simulink model "test_winds"  (R2014b)
settings: Solver=ode45  StartTime=0.0  StopTime=10.0  RelTol=1e-3
values from neighbouring files (symbols this model uses):
  TestInputs =     [unit_test_inputs.mat]
libraries: simulink_extras x10, simulink x2, csu_afm_aerodynamics_lib x1
settings Model: Creator=gnc  LastModifiedBy=mstewart
settings DebuggingCC: UnderspecifiedInitializationDetection=Classic  MergeDetectMultiDrivingBlocksExec=none  SolverPrmCheckMsg=none

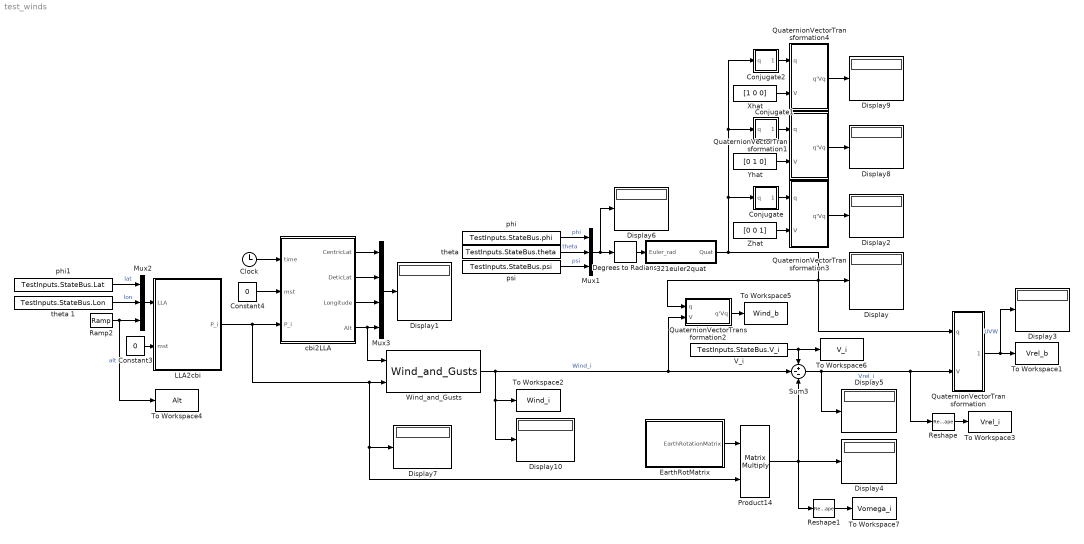
== system test_winds ==
  321euler2quat : Subsystem
  Clock : Clock
  Conjugate : Subsystem
  Conjugate1 : Subsystem
  Conjugate2 : Subsystem
  Constant3 : Constant  Value=0
  Constant4 : Constant  Value=0
  Degrees to Radians : simulink_extras/Transformations/Degrees to Radians
  Display{,1..10} (11 alike) : Display
  EarthRotMatrix : Subsystem
  LLA2cbi : Subsystem  mask(LLA to ECI Conversion){a=6378137.0, flatten=1/298.257223563}
      mask prompts: a "Central Body Semi-major Axis, a [m]"; flatten "Central Body Flattening Parameter, flatten [ND]"
      mask help: Converts Geodetic Latitude, Longitude, and Altitude into Central Body Inertial Coordinates. Inputs are [deg deg m]. Output is in [m]eters.
  Mux1 : Mux  Inputs=3
  Mux2 : Mux  Inputs=3
  Mux3 : Mux
  Product14 : Product  Multiplication=Matrix(*)  SaturateOnIntegerOverflow=on  OutDataTypeStr=Inherit: Same as first input
  QuaternionVectorTransformation : Subsystem
  QuaternionVectorTransformation1 : Subsystem
  QuaternionVectorTransformation2 : Subsystem
  QuaternionVectorTransformation3 : Subsystem
  QuaternionVectorTransformation4 : Subsystem
  Ramp2 : simulink/Sources/Ramp  slope=TestInputs.StateBus.AltDot  start=0  X0=TestInputs.StateBus.Alt
  Reshape : Reshape
  Reshape1 : Reshape
  Sum3 : Sum  Inputs=+--
  To Workspace1 : ToWorkspace  VariableName=Vrel_b  SaveFormat=Timeseries  SampleTime=-1
  To Workspace2 : ToWorkspace  VariableName=Wind_i  SaveFormat=Timeseries  SampleTime=-1
  To Workspace3 : ToWorkspace  VariableName=Vrel_i  SaveFormat=Timeseries  SampleTime=-1
  To Workspace4 : ToWorkspace  VariableName=Alt  SaveFormat=Timeseries  SampleTime=-1
  To Workspace5 : ToWorkspace  VariableName=Wind_b  SaveFormat=Timeseries  SampleTime=-1
  To Workspace6 : ToWorkspace  VariableName=V_i  SaveFormat=Timeseries  SampleTime=-1
  To Workspace7 : ToWorkspace  VariableName=Vomega_i  SaveFormat=Timeseries  SampleTime=-1
  V_i : Constant  Value=TestInputs.StateBus.V_i  VectorParams1D=off
  Wind_and_Gusts : csu_afm_aerodynamics_lib/csu_afm_aerodynamics/Wind_and_Gusts  SystemSampleTime=-1
  Xhat : Constant  Value=[1 0 0]
  Yhat : Constant  Value=[0 1 0]
  Zhat : Constant  Value=[0 0 1]
  cbi2LLA : Subsystem  mask{a=6378137.0, flatten=1/298.257223563, omega=7.2921151467e-5}
      mask prompts: a "Central Body Semi-major Axis, a [m]"; flatten "Central Body Flattening Parameter, flatten [ND]"; omega "Central Body Rotation Rate, omega [rad/s]"
      mask help:
      | % FUNCTION cbi2lla
      | %   Compute Detic Latitude, Centric Latitude, Longitude, and Detic Altitude
      | %   from Central Body Inertial Coordinates
      | %
      | %   [latD, latC, lon, alt]  = cbi2lla( P_i, mst)
      | %
      | %  INPUTS
      | %   P_i         [1x3]   {m}         Position in Central Body Inertial Frame
      | %   mst         [1x1]   (degrees)   Mean Sidereal Time
      | %
      | %  OUTPUTS
      | %   latD        [1x1]   {deg}       Detic Latitude
      | %   latC        [1x1]   {deg}       Centric Latitude
      | %   lon         [1x1]   {deg}       Longitude
      | %   alt         [1x1]   {m}         Detic Altitude
      | %
      | %  SOURCE
      | %   Borkowski, K.M. "Accurate Algorithms to Transform Geocentric to
      | %   Geodetic Coordinates"  Torun Radio Astronomy Observatory, Nicolaus
      | %   Copernicaus University, ul. Chopina 12/18, PL-87-100 Torun, Poland
      | %   Bullentin Geodesique, 63 (1989), pp. 50-56
      | %     http://www.astro.uni.torun.pl/~kb/Papers/geod/Geod-BG.htm
  phi : Constant  Value=TestInputs.StateBus.phi  VectorParams1D=off
  phi1 : Constant  Value=TestInputs.StateBus.Lat  VectorParams1D=off
  psi : Constant  Value=TestInputs.StateBus.psi  VectorParams1D=off
  "theta " : Constant  Value=TestInputs.StateBus.theta  VectorParams1D=off
  theta 1 : Constant  Value=TestInputs.StateBus.Lon  VectorParams1D=off
  wires:
  Wind_and_Gusts/1 -> Sum3/2, QuaternionVectorTransformation2/2(V), To Workspace2/1, Display10/1  "Wind_i"
  cbi2LLA/4(Alt) -> Wind_and_Gusts/1, Mux3/4
  QuaternionVectorTransformation/1(q'Vq) -> Display3/1, To Workspace1/1  "UVW"
  Sum3/1 -> Display5/1, Reshape/1, QuaternionVectorTransformation/2(V)  "Vrel_i"
  LLA2cbi/1(P_i) -> cbi2LLA/3(P_i), Wind_and_Gusts/2, Display7/1, Product14/2
  EarthRotMatrix/1(EarthRotationMatrix) -> Product14/1
  Reshape/1 -> To Workspace3/1
  phi/1 -> Mux1/1  "phi"
  "theta "/1 -> Mux1/2  "theta"
  Mux1/1 -> Display6/1, Degrees to Radians/1
  Degrees to Radians/1 -> 321euler2quat/1(Euler_rad)
  psi/1 -> Mux1/3  "psi"
  Product14/1 -> Reshape1/1, Sum3/3, Display4/1
  QuaternionVectorTransformation2/1(q'Vq) -> To Workspace5/1
  cbi2LLA/1(CentricLat) -> Mux3/1
  cbi2LLA/2(DeticLat) -> Mux3/2
  cbi2LLA/3(Longitude) -> Mux3/3
  Constant4/1 -> cbi2LLA/2(mst)
  Clock/1 -> cbi2LLA/1(time)
  Constant3/1 -> LLA2cbi/2(mst)
  Mux2/1 -> LLA2cbi/1(LLA)
  theta 1/1 -> Mux2/2  "lon"
  Ramp2/1 -> To Workspace4/1, Mux2/3  "alt"
  phi1/1 -> Mux2/1  "lat"
  Mux3/1 -> Display1/1
  Zhat/1 -> QuaternionVectorTransformation3/2(V)
  QuaternionVectorTransformation3/1(q'Vq) -> Display2/1
  V_i/1 -> To Workspace6/1, Sum3/1
  321euler2quat/1(Quat) -> Conjugate2/1(q), Conjugate1/1(q), Conjugate/1(q), QuaternionVectorTransformation/1(q), QuaternionVectorTransformation2/1(q), Display/1
  Conjugate/1(q') -> QuaternionVectorTransformation3/1(q)
  Yhat/1 -> QuaternionVectorTransformation1/2(V)
  QuaternionVectorTransformation1/1(q'Vq) -> Display8/1
  Conjugate1/1(q') -> QuaternionVectorTransformation1/1(q)
  Xhat/1 -> QuaternionVectorTransformation4/2(V)
  QuaternionVectorTransformation4/1(q'Vq) -> Display9/1
  Conjugate2/1(q') -> QuaternionVectorTransformation4/1(q)
  Reshape1/1 -> To Workspace7/1

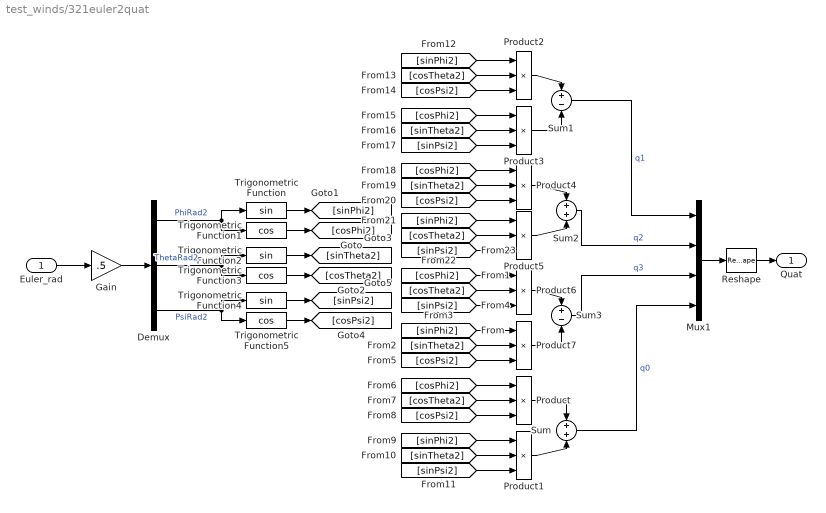
== system test_winds/321euler2quat ==
  Euler_rad : Inport
  Demux : Demux  Outputs=3
  Gain : Gain  Gain=.5
  Mux1 : Mux
  Product{,1..7} (8 alike) : Product  Inputs=3  RndMeth=Zero
  Reshape : Reshape
  Sum : Sum  Inputs=+|+
  Sum1 : Sum  Inputs=+|-
  Sum2 : Sum  Inputs=+|+
  Sum3 : Sum  Inputs=+|-
  Trigonometric Function : Trigonometry
  Trigonometric Function1 : Trigonometry  Operator=cos
  Trigonometric Function2 : Trigonometry
  Trigonometric Function3 : Trigonometry  Operator=cos
  Trigonometric Function4 : Trigonometry
  Trigonometric Function5 : Trigonometry  Operator=cos
  Quat : Outport
  wires:
  Reshape/1 -> Quat/1
  Mux1/1 -> Reshape/1
  Euler_rad/1 -> Gain/1
  [cosPsi2] -> Product7/3
  [sinTheta2] -> Product7/2
  [sinPhi2] -> Product7/1
  [sinPsi2] -> Product6/3
  [cosTheta2] -> Product6/2
  [cosPhi2] -> Product6/1
  Product6/1 -> Sum3/1
  Product7/1 -> Sum3/2
  Product5/1 -> Sum2/2
  [sinPsi2] -> Product5/3
  [cosTheta2] -> Product5/2
  [sinPhi2] -> Product5/1
  Product4/1 -> Sum2/1
  [cosPsi2] -> Product4/3
  [sinTheta2] -> Product4/2
  [cosPhi2] -> Product4/1
  Product3/1 -> Sum1/2
  [sinPsi2] -> Product3/3
  [sinTheta2] -> Product3/2
  [cosPhi2] -> Product3/1
  Product2/1 -> Sum1/1
  [cosPsi2] -> Product2/3
  [cosTheta2] -> Product2/2
  [sinPhi2] -> Product2/1
  [sinPsi2] -> Product1/3
  [sinTheta2] -> Product1/2
  [sinPhi2] -> Product1/1
  Product1/1 -> Sum/2
  Product/1 -> Sum/1
  [cosPsi2] -> Product/3
  [cosTheta2] -> Product/2
  [cosPhi2] -> Product/1
  Trigonometric Function5/1 -> [cosPsi2]
  Trigonometric Function4/1 -> [sinPsi2]
  Trigonometric Function3/1 -> [cosTheta2]
  Trigonometric Function2/1 -> [sinTheta2]
  Trigonometric Function1/1 -> [cosPhi2]
  Trigonometric Function/1 -> [sinPhi2]
  Demux/3 -> Trigonometric Function5/1, Trigonometric Function4/1  "PsiRad2"
  Demux/2 -> Trigonometric Function3/1, Trigonometric Function2/1  "ThetaRad2"
  Demux/1 -> Trigonometric Function1/1, Trigonometric Function/1  "PhiRad2"
  Gain/1 -> Demux/1
  Sum1/1 -> Mux1/1  "q1"
  Sum2/1 -> Mux1/2  "q2"
  Sum3/1 -> Mux1/3  "q3"
  Sum/1 -> Mux1/4  "q0"

== system test_winds/Conjugate ==
  q : Inport  PortDimensions=4
  Demux : Demux  Outputs=[3 1]
  Gain : Gain  Gain=-1  SaturateOnIntegerOverflow=on  OutDataTypeStr=Inherit: Same as input  ParamDataTypeStr=Inherit: Same as input
  Mux : Mux  Inputs=2
  q' : Outport  InitialOutput=0
  wires:
  Mux/1 -> q'/1
  Demux/2 -> Mux/2  "q(4)"
  Gain/1 -> Mux/1
  Demux/1 -> Gain/1  "[ q(1)  q(2)  q(3) ]"
  q/1 -> Demux/1

== system test_winds/Conjugate1 ==
  q : Inport  PortDimensions=4
  Demux : Demux  Outputs=[3 1]
  Gain : Gain  Gain=-1  SaturateOnIntegerOverflow=on  OutDataTypeStr=Inherit: Same as input  ParamDataTypeStr=Inherit: Same as input
  Mux : Mux  Inputs=2
  q' : Outport  InitialOutput=0
  wires:
  q/1 -> Demux/1
  Demux/1 -> Gain/1  "[ q(1)  q(2)  q(3) ]"
  Gain/1 -> Mux/1
  Demux/2 -> Mux/2  "q(4)"
  Mux/1 -> q'/1

== system test_winds/Conjugate2 ==
  q : Inport  PortDimensions=4
  Demux : Demux  Outputs=[3 1]
  Gain : Gain  Gain=-1  SaturateOnIntegerOverflow=on  OutDataTypeStr=Inherit: Same as input  ParamDataTypeStr=Inherit: Same as input
  Mux : Mux  Inputs=2
  q' : Outport  InitialOutput=0
  wires:
  q/1 -> Demux/1
  Demux/1 -> Gain/1  "[ q(1)  q(2)  q(3) ]"
  Gain/1 -> Mux/1
  Demux/2 -> Mux/2  "q(4)"
  Mux/1 -> q'/1

== system test_winds/EarthRotMatrix ==
  Constant{1..7} (7 alike) : Constant  Value=0
  EarthRate : Constant  Value=7.2921151467e-5
  Gain1 : Gain  Gain=-1  SaturateOnIntegerOverflow=on  OutDataTypeStr=Inherit: Same as input  ParamDataTypeStr=Inherit: Same as input
  Matrix Concatenation : Concatenate  NumInputs=3  Mode=Multidimensional array  ConcatenateDimension=2
  Mux : Mux  Inputs=3
  Mux1 : Mux  Inputs=3
  Mux2 : Mux  Inputs=3
  EarthRotationMatrix : Outport
  wires:
  Mux2/1 -> Matrix Concatenation/3
  Matrix Concatenation/1 -> EarthRotationMatrix/1
  EarthRate/1 -> [omegaE]
  [omegaE] -> Mux/2
  Constant5/1 -> Mux/1
  Constant6/1 -> Mux/3
  Constant4/1 -> Mux1/2
  Constant7/1 -> Mux2/3
  Constant3/1 -> Mux2/2
  Constant1/1 -> Mux2/1
  Constant2/1 -> Mux1/3
  Gain1/1 -> Mux1/1
  Mux1/1 -> Matrix Concatenation/2
  Mux/1 -> Matrix Concatenation/1
  [omegaE] -> Gain1/1

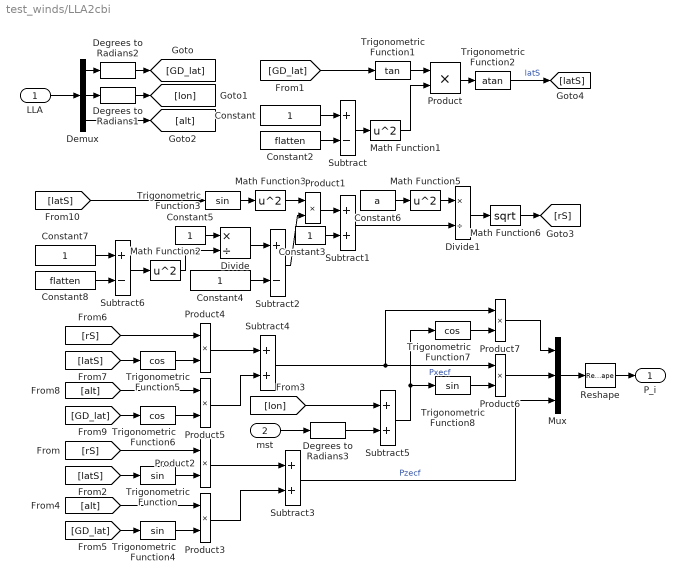
== system test_winds/LLA2cbi ==
  LLA : Inport
  mst : Inport  Port=2
  Constant{,3..5,7} (5 alike) : Constant
  Constant2 : Constant  Value=flatten
  Constant6 : Constant  Value=a
  Constant8 : Constant  Value=flatten
  Degrees to Radians1 : simulink_extras/Transformations/Degrees to Radians
  Degrees to Radians2 : simulink_extras/Transformations/Degrees to Radians
  Degrees to Radians3 : simulink_extras/Transformations/Degrees to Radians
  Demux : Demux  Outputs=3
  Divide : Product  Inputs=*/
  Divide1 : Product  Inputs=*/
  Math Function{1..3,5} (4 alike) : Math  Operator=square  SaturateOnIntegerOverflow=on
  Math Function6 : Math  Operator=sqrt  SaturateOnIntegerOverflow=on
  Mux : Mux  Inputs=3
  Product{,1..7} (8 alike) : Product  RndMeth=Zero
  Reshape : Reshape  OutputDimensionality=Column vector (2-D)
  Subtract : Sum  Inputs=+-
  Subtract{1,3..5} (4 alike) : Sum
  Subtract2 : Sum  Inputs=+-
  Subtract6 : Sum  Inputs=+-
  Trigonometric Function{,3..4,8} (4 alike) : Trigonometry
  Trigonometric Function1 : Trigonometry  Operator=tan
  Trigonometric Function2 : Trigonometry  Operator=atan
  Trigonometric Function5 : Trigonometry  Operator=cos
  Trigonometric Function6 : Trigonometry  Operator=cos
  Trigonometric Function7 : Trigonometry  Operator=cos
  P_i : Outport
  wires:
  Math Function2/1 -> Divide/2
  Subtract6/1 -> Math Function2/1
  Constant8/1 -> Subtract6/2
  Constant7/1 -> Subtract6/1
  [latS] -> Trigonometric Function3/1
  Trigonometric Function2/1 -> [latS]  "latS"
  Product6/1 -> Mux/2
  Product7/1 -> Mux/1
  Trigonometric Function7/1 -> Product7/2
  Trigonometric Function8/1 -> Product6/2
  Subtract4/1 -> Product7/1, Product6/1  "Pxecf"
  Subtract5/1 -> Trigonometric Function7/1, Trigonometric Function8/1
  [lon] -> Subtract5/1
  Degrees to Radians3/1 -> Subtract5/2
  mst/1 -> Degrees to Radians3/1
  Trigonometric Function6/1 -> Product5/2
  [alt] -> Product5/1
  Trigonometric Function5/1 -> Product4/2
  [rS] -> Product4/1
  Product5/1 -> Subtract4/2
  [GD_lat] -> Trigonometric Function6/1
  Product4/1 -> Subtract4/1
  [latS] -> Trigonometric Function5/1
  Mux/1 -> Reshape/1
  Subtract3/1 -> Mux/3  "Pzecf"
  Trigonometric Function4/1 -> Product3/2
  [alt] -> Product3/1
  Trigonometric Function/1 -> Product2/2
  [rS] -> Product2/1
  Product3/1 -> Subtract3/2
  [GD_lat] -> Trigonometric Function4/1
  Product2/1 -> Subtract3/1
  [latS] -> Trigonometric Function/1
  Math Function6/1 -> [rS]
  Divide1/1 -> Math Function6/1
  Math Function5/1 -> Divide1/1
  Subtract1/1 -> Divide1/2
  Constant6/1 -> Math Function5/1
  Product1/1 -> Subtract1/1
  Math Function3/1 -> Product1/1
  Subtract2/1 -> Product1/2
  Divide/1 -> Subtract2/1
  Constant5/1 -> Divide/1
  Constant4/1 -> Subtract2/2
  Trigonometric Function3/1 -> Math Function3/1
  Product/1 -> Trigonometric Function2/1
  Trigonometric Function1/1 -> Product/1
  [GD_lat] -> Trigonometric Function1/1
  Constant3/1 -> Subtract1/2
  Math Function1/1 -> Product/2
  Subtract/1 -> Math Function1/1
  Constant2/1 -> Subtract/2
  Constant/1 -> Subtract/1
  Degrees to Radians1/1 -> [lon]
  Degrees to Radians2/1 -> [GD_lat]
  Demux/3 -> [alt]
  Demux/2 -> Degrees to Radians1/1
  Demux/1 -> Degrees to Radians2/1
  LLA/1 -> Demux/1
  Reshape/1 -> P_i/1

== system test_winds/QuaternionVectorTransformation ==
  q : Inport  PortDimensions=4
  V : Inport  Port=2  PortDimensions=3
  Constant : Constant  Value=0
  Mux : Mux  Inputs=2
  Quaternion Conjugate : Subsystem
  Quaternion Multiply : Subsystem
  Quaternion Multiply1 : Subsystem
  Selector : Selector  InputPortWidth=4  Indices=[1 2 3]
  q'Vq : Outport  InitialOutput=0
  wires:
  Selector/1 -> q'Vq/1
  V/1 -> Mux/1
  Constant/1 -> Mux/2
  q/1 -> Quaternion Multiply1/2(q2), Quaternion Conjugate/1(q)
  Quaternion Multiply1/1(q1q2) -> Selector/1
  Mux/1 -> Quaternion Multiply/2(q2)
  Quaternion Conjugate/1(q') -> Quaternion Multiply/1(q1)
  Quaternion Multiply/1(q1q2) -> Quaternion Multiply1/1(q1)

== system test_winds/QuaternionVectorTransformation1 ==
  q : Inport  PortDimensions=4
  V : Inport  Port=2  PortDimensions=3
  Constant : Constant  Value=0
  Mux : Mux  Inputs=2
  Quaternion Conjugate : Subsystem
  Quaternion Multiply : Subsystem
  Quaternion Multiply1 : Subsystem
  Selector : Selector  InputPortWidth=4  Indices=[1 2 3]
  q'Vq : Outport  InitialOutput=0
  wires:
  Selector/1 -> q'Vq/1
  V/1 -> Mux/1
  Constant/1 -> Mux/2
  q/1 -> Quaternion Multiply1/2(q2), Quaternion Conjugate/1(q)
  Quaternion Multiply1/1(q1q2) -> Selector/1
  Mux/1 -> Quaternion Multiply/2(q2)
  Quaternion Conjugate/1(q') -> Quaternion Multiply/1(q1)
  Quaternion Multiply/1(q1q2) -> Quaternion Multiply1/1(q1)

== system test_winds/QuaternionVectorTransformation2 ==
  q : Inport  PortDimensions=4
  V : Inport  Port=2  PortDimensions=3
  Constant : Constant  Value=0
  Mux : Mux  Inputs=2
  Quaternion Conjugate : Subsystem
  Quaternion Multiply : Subsystem
  Quaternion Multiply1 : Subsystem
  Selector : Selector  InputPortWidth=4  Indices=[1 2 3]
  q'Vq : Outport  InitialOutput=0
  wires:
  Quaternion Multiply/1(q1q2) -> Quaternion Multiply1/1(q1)
  Quaternion Conjugate/1(q') -> Quaternion Multiply/1(q1)
  Mux/1 -> Quaternion Multiply/2(q2)
  Quaternion Multiply1/1(q1q2) -> Selector/1
  q/1 -> Quaternion Conjugate/1(q), Quaternion Multiply1/2(q2)
  Constant/1 -> Mux/2
  V/1 -> Mux/1
  Selector/1 -> q'Vq/1

== system test_winds/QuaternionVectorTransformation3 ==
  q : Inport  PortDimensions=4
  V : Inport  Port=2  PortDimensions=3
  Constant : Constant  Value=0
  Mux : Mux  Inputs=2
  Quaternion Conjugate : Subsystem
  Quaternion Multiply : Subsystem
  Quaternion Multiply1 : Subsystem
  Selector : Selector  InputPortWidth=4  Indices=[1 2 3]
  q'Vq : Outport  InitialOutput=0
  wires:
  Quaternion Multiply/1(q1q2) -> Quaternion Multiply1/1(q1)
  Quaternion Conjugate/1(q') -> Quaternion Multiply/1(q1)
  Mux/1 -> Quaternion Multiply/2(q2)
  Quaternion Multiply1/1(q1q2) -> Selector/1
  q/1 -> Quaternion Conjugate/1(q), Quaternion Multiply1/2(q2)
  Constant/1 -> Mux/2
  V/1 -> Mux/1
  Selector/1 -> q'Vq/1

== system test_winds/QuaternionVectorTransformation4 ==
  q : Inport  PortDimensions=4
  V : Inport  Port=2  PortDimensions=3
  Constant : Constant  Value=0
  Mux : Mux  Inputs=2
  Quaternion Conjugate : Subsystem
  Quaternion Multiply : Subsystem
  Quaternion Multiply1 : Subsystem
  Selector : Selector  InputPortWidth=4  Indices=[1 2 3]
  q'Vq : Outport  InitialOutput=0
  wires:
  Selector/1 -> q'Vq/1
  V/1 -> Mux/1
  Constant/1 -> Mux/2
  q/1 -> Quaternion Multiply1/2(q2), Quaternion Conjugate/1(q)
  Quaternion Multiply1/1(q1q2) -> Selector/1
  Mux/1 -> Quaternion Multiply/2(q2)
  Quaternion Conjugate/1(q') -> Quaternion Multiply/1(q1)
  Quaternion Multiply/1(q1q2) -> Quaternion Multiply1/1(q1)

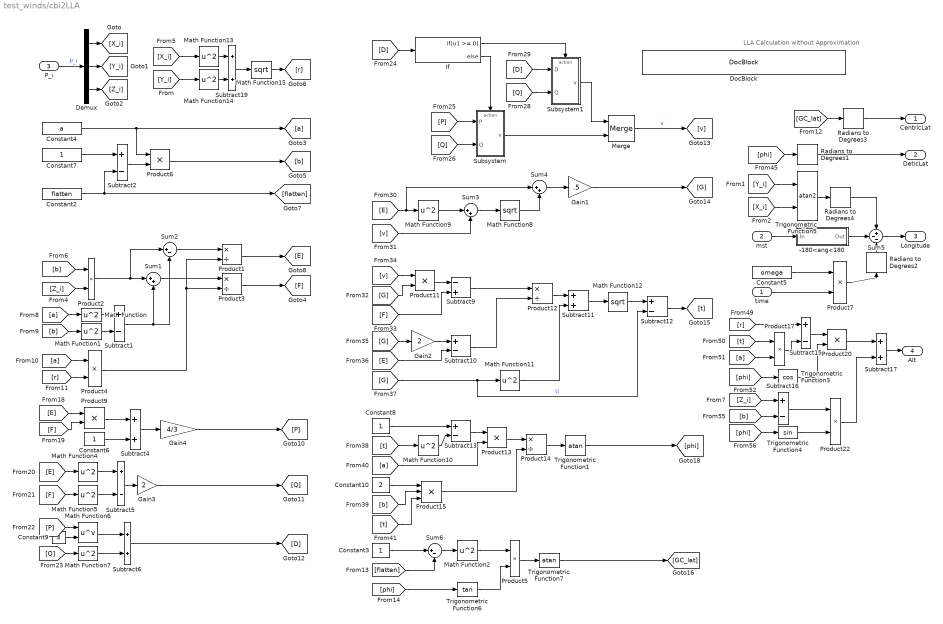
== system test_winds/cbi2LLA ==
  note: LLA Calculation without Approximation
  time : Inport
  mst : Inport  Port=2
  P_i : Inport  Port=3
  -180<ang<180 : Subsystem
  Constant10 : Constant  Value=2
  Constant2 : Constant  Value=flatten
  Constant{3,6..8} (4 alike) : Constant
  Constant4 : Constant  Value=a
  Constant5 : Constant  Value=omega
  Constant9 : Constant  Value=3
  Demux : Demux  Outputs=3
  DocBlock : simulink/Model-Wide Utilities/DocBlock  DocumentType=Text
      content=|
      | function [latD, latC, lon, alt]  = cbi2lla( P_i, mst)
      | % FUNCTION cbi2lla
      | %   Compute Detic Latitude, Centric Latitude, Longitude, and Detic Altitude
      | %   from Central Body Inertial Coordinates
      | %
      | %   [latD, latC, lon, alt]  = cbi2lla( P_i, mst)
      | %
      | %  INPUTS
      | %   P_i         [1x3]   {m}         Position in Central Body Inertial Frame
      | %   mst         [1x1]   (degrees)   Mean Sidereal Time
      | %
      | %  OUTPUTS
      | %   detic_lat   [1x1]   {deg}       Detic Latitude
      | %   centric_lat [1x1]   {deg}       Centric Latitude
      | %   lon         [1x1]   {deg}       Longitude
      | %   alt         [1x1]   {m}         Detic Altitude
      | %
      | %  SOURCE
      | %   Borkowski, K.M. "Accurate Algorithms to Transform Geocentric to
      | %   Geodetic Coordinates"  Torun Radio Astronomy Observatory, Nicolaus
      | %   Copernicaus University, ul. Chopina 12/18, PL-87-100 Torun, Poland
      | %   Bullentin Geodesique, 63 (1989), pp. 50-56
      | %     http://www.astro.uni.torun.pl/~kb/Papers/geod/Geod-BG.htm
      |
      | %% Constants
      | R2D = 180.0/acos(-1);
      | D2R = acos(-1)/180.0;
      |
      | X = P_i(1);
      | Y = P_i(2);
      | Z = P_i(3);
      |
      | %% Compute Detic Latitude & Detic Altitude ==========================
      | r = sqrt( X*X + Y*Y );
      | if (Z < 0)
      |     b = -b;
      | end
      |
      | E = ((b*Z) - (a*a - b*b))/(a*r);        % {Eq 10}
      | F = ((b*Z) + (a*a - b*b))/(a*r);        % {Eq 11}
      |
      | P = (4/3)*(E*F + 1);                    % {Eq 16}
      | Q = 2*(E*E - F*F);                      % {Eq 17}
      |
      | D = (P*P*P) + (Q*Q);                    % {Eq 15}
      | if (D < 0)
      |     v = 2*(sqrt(-P))*cos( (1/2)*acos(Q/((-P)^(3/2))) );     % {Eq 14b}
      | else
      |     v = ((sqrt(D) - Q)^(1/3)) - ((sqrt(D) + Q)^(1/3));      % {Eq 14a}
      | end
      |
      | G = (sqrt(E*E + v) + E)/2;              % {Eq 13}
      | t = sqrt( G*G + (F-v*G)/(2*G-E)) - G;   % {Eq 12}
      |
      | phi = atan( a*(1-t*t)/(2*b*t) );        % {Eq 18}
      | h = (r-a*t)*cos(phi) + (Z-b)*sin(phi);  % {Eq 19}
      |
      | latD = phi * R2D;
      | alt = h;
      |
      | %% Compute Longitude ======================================================
      | lon = atan( Y / X ) * R2D - mst;
      |
      | %% Compute Centric Latitude ============================================
      | %   Centric Latitude {deg}
      | latC = atan((1 - flatten)^2 * tan(latD * D2R)) * R2D;
  Gain1 : Gain  Gain=.5
  Gain2 : Gain  Gain=2
  Gain3 : Gain  Gain=2
  Gain4 : Gain  Gain=4/3
  If : If  IfExpression=u1 >= 0
  Math Function{,1..2,4..5,7,9..11,13..14} (11 alike) : Math  Operator=square  SaturateOnIntegerOverflow=on
  Math Function12 : Math  Operator=sqrt  SaturateOnIntegerOverflow=on
  Math Function15 : Math  Operator=sqrt  SaturateOnIntegerOverflow=on
  Math Function6 : Math  Operator=pow  SaturateOnIntegerOverflow=on
  Math Function8 : Math  Operator=sqrt  SaturateOnIntegerOverflow=on
  Merge : Merge
  Product{1,3,12,14} (4 alike) : Product  Inputs=*/  RndMeth=Zero
  Product{5..6,11,13,17,20,22} (7 alike) : Product  Inputs=**  RndMeth=Zero
  Product15 : Product  Inputs=***  RndMeth=Zero
  Product2 : Product  RndMeth=Zero
  Product4 : Product  RndMeth=Zero
  Product7 : Product  Inputs=**  SaturateOnIntegerOverflow=on  OutDataTypeStr=Inherit: Same as first input
  Product9 : Product  RndMeth=Zero
  Radians to Degrees{1..4} (4 alike) : simulink_extras/Transformations/Radians to Degrees
  Subsystem : Subsystem
  Subsystem1 : Subsystem
  Subtract{1..2,5,10,12..13,15..16} (8 alike) : Sum  Inputs=+-
  Subtract{4,6,11,17,19} (5 alike) : Sum
  Subtract9 : Sum  Inputs=-+
  Sum1 : Sum  Inputs=|++
  Sum2 : Sum  Inputs=|+-
  Sum3 : Sum  Inputs=|++
  Sum4 : Sum  Inputs=|++
  Sum5 : Sum  Inputs=+--
  Sum6 : Sum  Inputs=|+-
  Trigonometric Function1 : Trigonometry  Operator=atan
  Trigonometric Function3 : Trigonometry  Operator=cos
  Trigonometric Function4 : Trigonometry
  Trigonometric Function5 : Trigonometry  Operator=atan2
  Trigonometric Function6 : Trigonometry  Operator=tan
  Trigonometric Function7 : Trigonometry  Operator=atan
  CentricLat : Outport
  DeticLat : Outport  Port=2
  Longitude : Outport  Port=3
  Alt : Outport  Port=4
  wires:
  P_i/1 -> Demux/1  "P_i"
  [b] -> Product2/1
  [Z_i] -> Product2/2
  Product2/1 -> Sum1/1, Sum2/1
  [a] -> Math Function/1
  [b] -> Math Function1/1
  Math Function/1 -> Subtract1/1
  Math Function1/1 -> Subtract1/2
  Sum1/1 -> Product3/1
  [a] -> Product4/1
  [r] -> Product4/2
  Product4/1 -> Product3/2, Product1/2
  [E] -> Product9/1
  [F] -> Product9/2
  Constant6/1 -> Subtract4/2
  Product9/1 -> Subtract4/1
  Subtract4/1 -> Gain4/1
  [E] -> Math Function4/1
  [F] -> Math Function5/1
  Math Function4/1 -> Subtract5/1
  Math Function5/1 -> Subtract5/2
  Subtract5/1 -> Gain3/1
  Gain3/1 -> [Q]
  [P] -> Math Function6/1
  [Q] -> Math Function7/1
  Math Function6/1 -> Subtract6/1
  Math Function7/1 -> Subtract6/2
  Subtract6/1 -> [D]
  Constant9/1 -> Math Function6/2
  [D] -> If/1
  If/1 -> Subsystem1/Action
  If/2 -> Subsystem/Action
  [P] -> Subsystem/1(P)
  [Q] -> Subsystem/2(Q)
  [Q] -> Subsystem1/2(Q)
  [D] -> Subsystem1/1(D)
  Subsystem1/1(v) -> Merge/1
  Subsystem/1(v) -> Merge/2
  Merge/1 -> [v]  "v"
  [E] -> Math Function9/1, Sum4/1
  Math Function9/1 -> Sum3/1
  [v] -> Sum3/2
  Sum3/1 -> Math Function8/1
  Math Function8/1 -> Sum4/2
  Sum4/1 -> Gain1/1
  Gain1/1 -> [G]
  [G] -> Product11/2
  [v] -> Product11/1
  [F] -> Subtract9/2
  Product11/1 -> Subtract9/1
  Subtract9/1 -> Product12/1
  [G] -> Gain2/1
  Gain2/1 -> Subtract10/1
  [E] -> Subtract10/2
  Subtract10/1 -> Product12/2
  [G] -> Math Function11/1, Subtract12/2  "G"
  Product12/1 -> Subtract11/1
  Math Function11/1 -> Subtract11/2
  Subtract11/1 -> Math Function12/1
  Math Function12/1 -> Subtract12/1
  Subtract12/1 -> [t]
  [t] -> Math Function10/1
  Constant8/1 -> Subtract13/1
  Math Function10/1 -> Subtract13/2
  Subtract13/1 -> Product13/1
  [a] -> Product13/2
  Constant10/1 -> Product15/1
  [b] -> Product15/2
  [t] -> Product15/3
  Product15/1 -> Product14/2
  Product13/1 -> Product14/1
  Product14/1 -> Trigonometric Function1/1
  [phi] -> Radians to Degrees1/1
  Trigonometric Function1/1 -> [phi]
  [t] -> Product17/1
  [a] -> Product17/2
  [r] -> Subtract15/1
  Product17/1 -> Subtract15/2
  Radians to Degrees1/1 -> DeticLat/1
  [phi] -> Trigonometric Function3/1
  Subtract15/1 -> Product20/1
  Trigonometric Function3/1 -> Product20/2
  [b] -> Subtract16/2
  [Z_i] -> Subtract16/1
  [phi] -> Trigonometric Function4/1
  Subtract16/1 -> Product22/1
  Trigonometric Function4/1 -> Product22/2
  Product20/1 -> Subtract17/1
  Product22/1 -> Subtract17/2
  Subtract17/1 -> Alt/1
  Demux/1 -> [X_i]
  Demux/2 -> [Y_i]
  Demux/3 -> [Z_i]
  [X_i] -> Math Function13/1
  [Y_i] -> Math Function14/1
  Math Function13/1 -> Subtract19/1
  Math Function14/1 -> Subtract19/2
  Subtract19/1 -> Math Function15/1
  Math Function15/1 -> [r]
  Product1/1 -> [E]
  Product3/1 -> [F]
  Sum2/1 -> Product1/1
  Subtract1/1 -> Sum1/2, Sum2/2
  Gain4/1 -> [P]
  [X_i] -> Trigonometric Function5/2
  [Y_i] -> Trigonometric Function5/1
  [GC_lat] -> Radians to Degrees3/1
  Constant3/1 -> Sum6/1
  [flatten] -> Sum6/2
  Sum6/1 -> Math Function2/1
  [phi] -> Trigonometric Function6/1
  Math Function2/1 -> Product5/1
  Trigonometric Function6/1 -> Product5/2
  Product5/1 -> Trigonometric Function7/1
  Trigonometric Function7/1 -> [GC_lat]
  Radians to Degrees3/1 -> CentricLat/1
  Trigonometric Function5/1 -> Radians to Degrees4/1
  Radians to Degrees4/1 -> Sum5/1
  Sum5/1 -> Longitude/1
  Product7/1 -> Radians to Degrees2/1
  time/1 -> Product7/2
  Constant5/1 -> Product7/1
  Radians to Degrees2/1 -> Sum5/3
  mst/1 -> -180<ang<180/1(In)
  -180<ang<180/1(Out) -> Sum5/2
  Subtract2/1 -> Product6/2
  Constant2/1 -> Subtract2/2, [flatten]
  Constant7/1 -> Subtract2/1
  Constant4/1 -> Product6/1, [a]
  Product6/1 -> [b]

== system test_winds/QuaternionVectorTransformation/Quaternion Conjugate ==
  q : Inport  PortDimensions=4
  Demux : Demux  Outputs=[3 1]
  Gain : Gain  Gain=-1  SaturateOnIntegerOverflow=on  OutDataTypeStr=Inherit: Same as input  ParamDataTypeStr=Inherit: Same as input
  Mux : Mux  Inputs=2
  q' : Outport  InitialOutput=0
  wires:
  q/1 -> Demux/1
  Demux/1 -> Gain/1  "[ q(1)  q(2)  q(3) ]"
  Gain/1 -> Mux/1
  Demux/2 -> Mux/2  "q(4)"
  Mux/1 -> q'/1

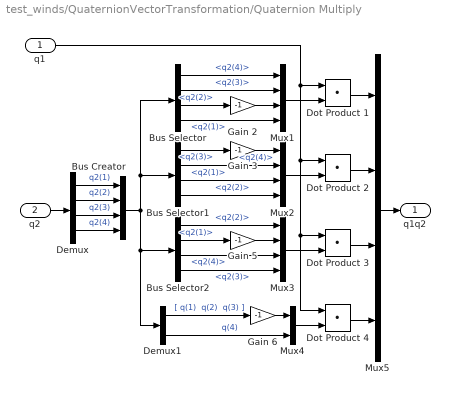
== system test_winds/QuaternionVectorTransformation/Quaternion Multiply ==
  q1 : Inport  PortDimensions=4
  q2 : Inport  Port=2  PortDimensions=4
  Bus Creator : BusCreator
  Bus Selector : BusSelector  OutputSignals=q2(4),q2(3),q2(2),q2(1)
  Bus Selector1 : BusSelector  OutputSignals=q2(3),q2(4),q2(1),q2(2)
  Bus Selector2 : BusSelector  OutputSignals=q2(2),q2(1),q2(4),q2(3)
  Demux : Demux
  Demux1 : Demux  Outputs=[3 1]
  Dot Product {1..4} (4 alike) : DotProduct  InputSameDT=on  OutDataTypeStr=Inherit: Inherit via internal rule
  Gain {2..3,5..6} (4 alike) : Gain  Gain=-1  SaturateOnIntegerOverflow=on  OutDataTypeStr=Inherit: Same as input  ParamDataTypeStr=Inherit: Same as input
  Mux{1..3,5} (4 alike) : Mux
  Mux4 : Mux  Inputs=2
  q1q2 : Outport  InitialOutput=0
  wires:
  Demux1/2 -> Mux4/2  "q(4)"
  Gain 6/1 -> Mux4/1
  Demux1/1 -> Gain 6/1  "[ q(1)  q(2)  q(3) ]"
  Mux4/1 -> Dot Product 4/2
  Bus Selector2/4 -> Mux3/4  "<q2(3)>"
  Bus Selector2/1 -> Mux3/1  "<q2(2)>"
  Gain 5/1 -> Mux3/2
  Bus Selector2/2 -> Gain 5/1  "<q2(1)>"
  Bus Selector1/4 -> Mux2/4  "<q2(2)>"
  Bus Selector1/3 -> Mux2/3  "<q2(1)>"
  Gain 3/1 -> Mux2/1
  Bus Selector1/1 -> Gain 3/1  "<q2(3)>"
  Bus Selector/4 -> Mux1/4  "<q2(1)>"
  Gain 2/1 -> Mux1/3
  Bus Selector/3 -> Gain 2/1  "<q2(2)>"
  Bus Selector/2 -> Mux1/2  "<q2(3)>"
  Bus Selector/1 -> Mux1/1  "<q2(4)>"
  Bus Selector1/2 -> Mux2/2  "<q2(4)>"
  Bus Selector2/3 -> Mux3/3  "<q2(4)>"
  Mux1/1 -> Dot Product 1/2
  Mux2/1 -> Dot Product 2/2
  Mux3/1 -> Dot Product 3/2
  q1/1 -> Dot Product 1/1, Dot Product 2/1, Dot Product 3/1, Dot Product 4/1
  Dot Product 1/1 -> Mux5/1
  Dot Product 3/1 -> Mux5/3
  Dot Product 4/1 -> Mux5/4
  Mux5/1 -> q1q2/1
  Dot Product 2/1 -> Mux5/2
  Bus Creator/1 -> Demux1/1, Bus Selector2/1, Bus Selector/1, Bus Selector1/1
  q2/1 -> Demux/1
  Demux/1 -> Bus Creator/1  "q2(1)"
  Demux/2 -> Bus Creator/2  "q2(2)"
  Demux/3 -> Bus Creator/3  "q2(3)"
  Demux/4 -> Bus Creator/4  "q2(4)"

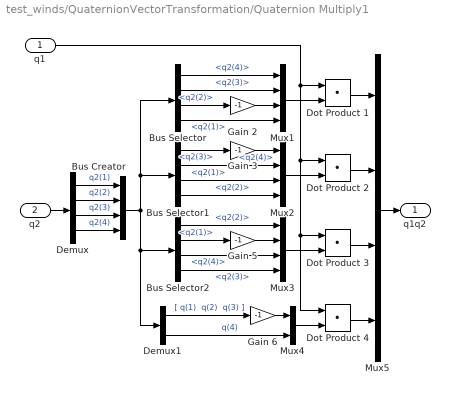
== system test_winds/QuaternionVectorTransformation/Quaternion Multiply1 ==
  q1 : Inport  PortDimensions=4
  q2 : Inport  Port=2  PortDimensions=4
  Bus Creator : BusCreator
  Bus Selector : BusSelector  OutputSignals=q2(4),q2(3),q2(2),q2(1)
  Bus Selector1 : BusSelector  OutputSignals=q2(3),q2(4),q2(1),q2(2)
  Bus Selector2 : BusSelector  OutputSignals=q2(2),q2(1),q2(4),q2(3)
  Demux : Demux
  Demux1 : Demux  Outputs=[3 1]
  Dot Product {1..4} (4 alike) : DotProduct  InputSameDT=on  OutDataTypeStr=Inherit: Inherit via internal rule
  Gain {2..3,5..6} (4 alike) : Gain  Gain=-1  SaturateOnIntegerOverflow=on  OutDataTypeStr=Inherit: Same as input  ParamDataTypeStr=Inherit: Same as input
  Mux{1..3,5} (4 alike) : Mux
  Mux4 : Mux  Inputs=2
  q1q2 : Outport  InitialOutput=0
  wires:
  Demux1/2 -> Mux4/2  "q(4)"
  Gain 6/1 -> Mux4/1
  Demux1/1 -> Gain 6/1  "[ q(1)  q(2)  q(3) ]"
  Mux4/1 -> Dot Product 4/2
  Bus Selector2/4 -> Mux3/4  "<q2(3)>"
  Bus Selector2/1 -> Mux3/1  "<q2(2)>"
  Gain 5/1 -> Mux3/2
  Bus Selector2/2 -> Gain 5/1  "<q2(1)>"
  Bus Selector1/4 -> Mux2/4  "<q2(2)>"
  Bus Selector1/3 -> Mux2/3  "<q2(1)>"
  Gain 3/1 -> Mux2/1
  Bus Selector1/1 -> Gain 3/1  "<q2(3)>"
  Bus Selector/4 -> Mux1/4  "<q2(1)>"
  Gain 2/1 -> Mux1/3
  Bus Selector/3 -> Gain 2/1  "<q2(2)>"
  Bus Selector/2 -> Mux1/2  "<q2(3)>"
  Bus Selector/1 -> Mux1/1  "<q2(4)>"
  Bus Selector1/2 -> Mux2/2  "<q2(4)>"
  Bus Selector2/3 -> Mux3/3  "<q2(4)>"
  Mux1/1 -> Dot Product 1/2
  Mux2/1 -> Dot Product 2/2
  Mux3/1 -> Dot Product 3/2
  q1/1 -> Dot Product 1/1, Dot Product 2/1, Dot Product 3/1, Dot Product 4/1
  Dot Product 1/1 -> Mux5/1
  Dot Product 3/1 -> Mux5/3
  Dot Product 4/1 -> Mux5/4
  Mux5/1 -> q1q2/1
  Dot Product 2/1 -> Mux5/2
  Bus Creator/1 -> Demux1/1, Bus Selector2/1, Bus Selector/1, Bus Selector1/1
  q2/1 -> Demux/1
  Demux/1 -> Bus Creator/1  "q2(1)"
  Demux/2 -> Bus Creator/2  "q2(2)"
  Demux/3 -> Bus Creator/3  "q2(3)"
  Demux/4 -> Bus Creator/4  "q2(4)"

== system test_winds/QuaternionVectorTransformation1/Quaternion Conjugate ==
  q : Inport  PortDimensions=4
  Demux : Demux  Outputs=[3 1]
  Gain : Gain  Gain=-1  SaturateOnIntegerOverflow=on  OutDataTypeStr=Inherit: Same as input  ParamDataTypeStr=Inherit: Same as input
  Mux : Mux  Inputs=2
  q' : Outport  InitialOutput=0
  wires:
  q/1 -> Demux/1
  Demux/1 -> Gain/1  "[ q(1)  q(2)  q(3) ]"
  Gain/1 -> Mux/1
  Demux/2 -> Mux/2  "q(4)"
  Mux/1 -> q'/1

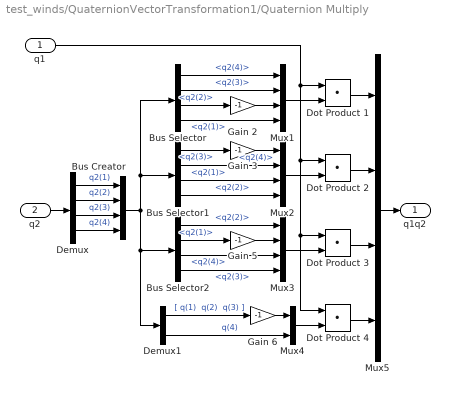
== system test_winds/QuaternionVectorTransformation1/Quaternion Multiply ==
  q1 : Inport  PortDimensions=4
  q2 : Inport  Port=2  PortDimensions=4
  Bus Creator : BusCreator
  Bus Selector : BusSelector  OutputSignals=q2(4),q2(3),q2(2),q2(1)
  Bus Selector1 : BusSelector  OutputSignals=q2(3),q2(4),q2(1),q2(2)
  Bus Selector2 : BusSelector  OutputSignals=q2(2),q2(1),q2(4),q2(3)
  Demux : Demux
  Demux1 : Demux  Outputs=[3 1]
  Dot Product {1..4} (4 alike) : DotProduct  InputSameDT=on  OutDataTypeStr=Inherit: Inherit via internal rule
  Gain {2..3,5..6} (4 alike) : Gain  Gain=-1  SaturateOnIntegerOverflow=on  OutDataTypeStr=Inherit: Same as input  ParamDataTypeStr=Inherit: Same as input
  Mux{1..3,5} (4 alike) : Mux
  Mux4 : Mux  Inputs=2
  q1q2 : Outport  InitialOutput=0
  wires:
  Demux1/2 -> Mux4/2  "q(4)"
  Gain 6/1 -> Mux4/1
  Demux1/1 -> Gain 6/1  "[ q(1)  q(2)  q(3) ]"
  Mux4/1 -> Dot Product 4/2
  Bus Selector2/4 -> Mux3/4  "<q2(3)>"
  Bus Selector2/1 -> Mux3/1  "<q2(2)>"
  Gain 5/1 -> Mux3/2
  Bus Selector2/2 -> Gain 5/1  "<q2(1)>"
  Bus Selector1/4 -> Mux2/4  "<q2(2)>"
  Bus Selector1/3 -> Mux2/3  "<q2(1)>"
  Gain 3/1 -> Mux2/1
  Bus Selector1/1 -> Gain 3/1  "<q2(3)>"
  Bus Selector/4 -> Mux1/4  "<q2(1)>"
  Gain 2/1 -> Mux1/3
  Bus Selector/3 -> Gain 2/1  "<q2(2)>"
  Bus Selector/2 -> Mux1/2  "<q2(3)>"
  Bus Selector/1 -> Mux1/1  "<q2(4)>"
  Bus Selector1/2 -> Mux2/2  "<q2(4)>"
  Bus Selector2/3 -> Mux3/3  "<q2(4)>"
  Mux1/1 -> Dot Product 1/2
  Mux2/1 -> Dot Product 2/2
  Mux3/1 -> Dot Product 3/2
  q1/1 -> Dot Product 1/1, Dot Product 2/1, Dot Product 3/1, Dot Product 4/1
  Dot Product 1/1 -> Mux5/1
  Dot Product 3/1 -> Mux5/3
  Dot Product 4/1 -> Mux5/4
  Mux5/1 -> q1q2/1
  Dot Product 2/1 -> Mux5/2
  Bus Creator/1 -> Demux1/1, Bus Selector2/1, Bus Selector/1, Bus Selector1/1
  q2/1 -> Demux/1
  Demux/1 -> Bus Creator/1  "q2(1)"
  Demux/2 -> Bus Creator/2  "q2(2)"
  Demux/3 -> Bus Creator/3  "q2(3)"
  Demux/4 -> Bus Creator/4  "q2(4)"

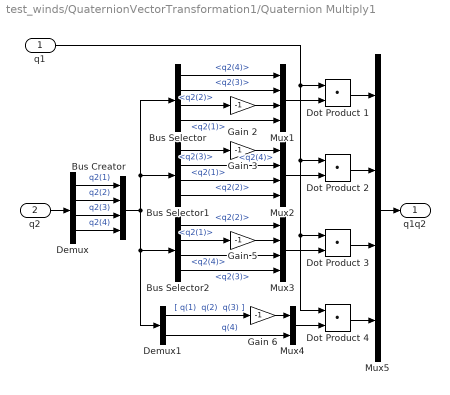
== system test_winds/QuaternionVectorTransformation1/Quaternion Multiply1 ==
  q1 : Inport  PortDimensions=4
  q2 : Inport  Port=2  PortDimensions=4
  Bus Creator : BusCreator
  Bus Selector : BusSelector  OutputSignals=q2(4),q2(3),q2(2),q2(1)
  Bus Selector1 : BusSelector  OutputSignals=q2(3),q2(4),q2(1),q2(2)
  Bus Selector2 : BusSelector  OutputSignals=q2(2),q2(1),q2(4),q2(3)
  Demux : Demux
  Demux1 : Demux  Outputs=[3 1]
  Dot Product {1..4} (4 alike) : DotProduct  InputSameDT=on  OutDataTypeStr=Inherit: Inherit via internal rule
  Gain {2..3,5..6} (4 alike) : Gain  Gain=-1  SaturateOnIntegerOverflow=on  OutDataTypeStr=Inherit: Same as input  ParamDataTypeStr=Inherit: Same as input
  Mux{1..3,5} (4 alike) : Mux
  Mux4 : Mux  Inputs=2
  q1q2 : Outport  InitialOutput=0
  wires:
  Demux1/2 -> Mux4/2  "q(4)"
  Gain 6/1 -> Mux4/1
  Demux1/1 -> Gain 6/1  "[ q(1)  q(2)  q(3) ]"
  Mux4/1 -> Dot Product 4/2
  Bus Selector2/4 -> Mux3/4  "<q2(3)>"
  Bus Selector2/1 -> Mux3/1  "<q2(2)>"
  Gain 5/1 -> Mux3/2
  Bus Selector2/2 -> Gain 5/1  "<q2(1)>"
  Bus Selector1/4 -> Mux2/4  "<q2(2)>"
  Bus Selector1/3 -> Mux2/3  "<q2(1)>"
  Gain 3/1 -> Mux2/1
  Bus Selector1/1 -> Gain 3/1  "<q2(3)>"
  Bus Selector/4 -> Mux1/4  "<q2(1)>"
  Gain 2/1 -> Mux1/3
  Bus Selector/3 -> Gain 2/1  "<q2(2)>"
  Bus Selector/2 -> Mux1/2  "<q2(3)>"
  Bus Selector/1 -> Mux1/1  "<q2(4)>"
  Bus Selector1/2 -> Mux2/2  "<q2(4)>"
  Bus Selector2/3 -> Mux3/3  "<q2(4)>"
  Mux1/1 -> Dot Product 1/2
  Mux2/1 -> Dot Product 2/2
  Mux3/1 -> Dot Product 3/2
  q1/1 -> Dot Product 1/1, Dot Product 2/1, Dot Product 3/1, Dot Product 4/1
  Dot Product 1/1 -> Mux5/1
  Dot Product 3/1 -> Mux5/3
  Dot Product 4/1 -> Mux5/4
  Mux5/1 -> q1q2/1
  Dot Product 2/1 -> Mux5/2
  Bus Creator/1 -> Demux1/1, Bus Selector2/1, Bus Selector/1, Bus Selector1/1
  q2/1 -> Demux/1
  Demux/1 -> Bus Creator/1  "q2(1)"
  Demux/2 -> Bus Creator/2  "q2(2)"
  Demux/3 -> Bus Creator/3  "q2(3)"
  Demux/4 -> Bus Creator/4  "q2(4)"

== system test_winds/QuaternionVectorTransformation2/Quaternion Conjugate ==
  q : Inport  PortDimensions=4
  Demux : Demux  Outputs=[3 1]
  Gain : Gain  Gain=-1  SaturateOnIntegerOverflow=on  OutDataTypeStr=Inherit: Same as input  ParamDataTypeStr=Inherit: Same as input
  Mux : Mux  Inputs=2
  q' : Outport  InitialOutput=0
  wires:
  Mux/1 -> q'/1
  Demux/2 -> Mux/2  "q(4)"
  Gain/1 -> Mux/1
  Demux/1 -> Gain/1  "[ q(1)  q(2)  q(3) ]"
  q/1 -> Demux/1

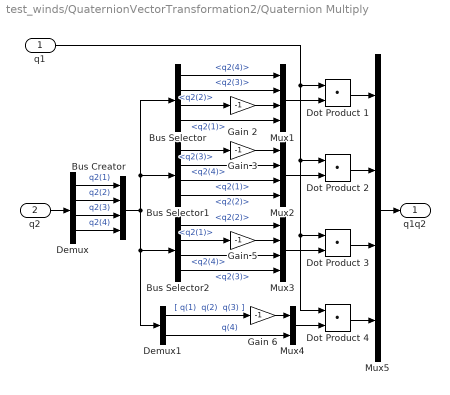
== system test_winds/QuaternionVectorTransformation2/Quaternion Multiply ==
  q1 : Inport  PortDimensions=4
  q2 : Inport  Port=2  PortDimensions=4
  Bus Creator : BusCreator
  Bus Selector : BusSelector  OutputSignals=q2(4),q2(3),q2(2),q2(1)
  Bus Selector1 : BusSelector  OutputSignals=q2(3),q2(4),q2(1),q2(2)
  Bus Selector2 : BusSelector  OutputSignals=q2(2),q2(1),q2(4),q2(3)
  Demux : Demux
  Demux1 : Demux  Outputs=[3 1]
  Dot Product {1..4} (4 alike) : DotProduct  InputSameDT=on  OutDataTypeStr=Inherit: Inherit via internal rule
  Gain {2..3,5..6} (4 alike) : Gain  Gain=-1  SaturateOnIntegerOverflow=on  OutDataTypeStr=Inherit: Same as input  ParamDataTypeStr=Inherit: Same as input
  Mux{1..3,5} (4 alike) : Mux
  Mux4 : Mux  Inputs=2
  q1q2 : Outport  InitialOutput=0
  wires:
  Demux/4 -> Bus Creator/4  "q2(4)"
  Demux/3 -> Bus Creator/3  "q2(3)"
  Demux/2 -> Bus Creator/2  "q2(2)"
  Demux/1 -> Bus Creator/1  "q2(1)"
  q2/1 -> Demux/1
  Bus Creator/1 -> Bus Selector1/1, Bus Selector/1, Bus Selector2/1, Demux1/1
  Dot Product 2/1 -> Mux5/2
  Mux5/1 -> q1q2/1
  Dot Product 4/1 -> Mux5/4
  Dot Product 3/1 -> Mux5/3
  Dot Product 1/1 -> Mux5/1
  q1/1 -> Dot Product 4/1, Dot Product 3/1, Dot Product 2/1, Dot Product 1/1
  Mux3/1 -> Dot Product 3/2
  Mux2/1 -> Dot Product 2/2
  Mux1/1 -> Dot Product 1/2
  Bus Selector2/3 -> Mux3/3  "<q2(4)>"
  Bus Selector1/2 -> Mux2/2  "<q2(4)>"
  Bus Selector/1 -> Mux1/1  "<q2(4)>"
  Bus Selector/2 -> Mux1/2  "<q2(3)>"
  Bus Selector/3 -> Gain 2/1  "<q2(2)>"
  Gain 2/1 -> Mux1/3
  Bus Selector/4 -> Mux1/4  "<q2(1)>"
  Bus Selector1/1 -> Gain 3/1  "<q2(3)>"
  Gain 3/1 -> Mux2/1
  Bus Selector1/3 -> Mux2/3  "<q2(1)>"
  Bus Selector1/4 -> Mux2/4  "<q2(2)>"
  Bus Selector2/2 -> Gain 5/1  "<q2(1)>"
  Gain 5/1 -> Mux3/2
  Bus Selector2/1 -> Mux3/1  "<q2(2)>"
  Bus Selector2/4 -> Mux3/4  "<q2(3)>"
  Mux4/1 -> Dot Product 4/2
  Demux1/1 -> Gain 6/1  "[ q(1)  q(2)  q(3) ]"
  Gain 6/1 -> Mux4/1
  Demux1/2 -> Mux4/2  "q(4)"

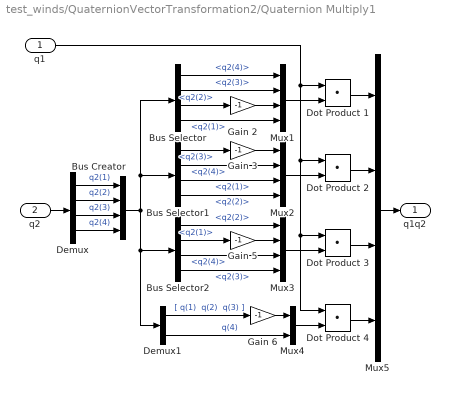
== system test_winds/QuaternionVectorTransformation2/Quaternion Multiply1 ==
  q1 : Inport  PortDimensions=4
  q2 : Inport  Port=2  PortDimensions=4
  Bus Creator : BusCreator
  Bus Selector : BusSelector  OutputSignals=q2(4),q2(3),q2(2),q2(1)
  Bus Selector1 : BusSelector  OutputSignals=q2(3),q2(4),q2(1),q2(2)
  Bus Selector2 : BusSelector  OutputSignals=q2(2),q2(1),q2(4),q2(3)
  Demux : Demux
  Demux1 : Demux  Outputs=[3 1]
  Dot Product {1..4} (4 alike) : DotProduct  InputSameDT=on  OutDataTypeStr=Inherit: Inherit via internal rule
  Gain {2..3,5..6} (4 alike) : Gain  Gain=-1  SaturateOnIntegerOverflow=on  OutDataTypeStr=Inherit: Same as input  ParamDataTypeStr=Inherit: Same as input
  Mux{1..3,5} (4 alike) : Mux
  Mux4 : Mux  Inputs=2
  q1q2 : Outport  InitialOutput=0
  wires:
  Demux/4 -> Bus Creator/4  "q2(4)"
  Demux/3 -> Bus Creator/3  "q2(3)"
  Demux/2 -> Bus Creator/2  "q2(2)"
  Demux/1 -> Bus Creator/1  "q2(1)"
  q2/1 -> Demux/1
  Bus Creator/1 -> Bus Selector1/1, Bus Selector/1, Bus Selector2/1, Demux1/1
  Dot Product 2/1 -> Mux5/2
  Mux5/1 -> q1q2/1
  Dot Product 4/1 -> Mux5/4
  Dot Product 3/1 -> Mux5/3
  Dot Product 1/1 -> Mux5/1
  q1/1 -> Dot Product 4/1, Dot Product 3/1, Dot Product 2/1, Dot Product 1/1
  Mux3/1 -> Dot Product 3/2
  Mux2/1 -> Dot Product 2/2
  Mux1/1 -> Dot Product 1/2
  Bus Selector2/3 -> Mux3/3  "<q2(4)>"
  Bus Selector1/2 -> Mux2/2  "<q2(4)>"
  Bus Selector/1 -> Mux1/1  "<q2(4)>"
  Bus Selector/2 -> Mux1/2  "<q2(3)>"
  Bus Selector/3 -> Gain 2/1  "<q2(2)>"
  Gain 2/1 -> Mux1/3
  Bus Selector/4 -> Mux1/4  "<q2(1)>"
  Bus Selector1/1 -> Gain 3/1  "<q2(3)>"
  Gain 3/1 -> Mux2/1
  Bus Selector1/3 -> Mux2/3  "<q2(1)>"
  Bus Selector1/4 -> Mux2/4  "<q2(2)>"
  Bus Selector2/2 -> Gain 5/1  "<q2(1)>"
  Gain 5/1 -> Mux3/2
  Bus Selector2/1 -> Mux3/1  "<q2(2)>"
  Bus Selector2/4 -> Mux3/4  "<q2(3)>"
  Mux4/1 -> Dot Product 4/2
  Demux1/1 -> Gain 6/1  "[ q(1)  q(2)  q(3) ]"
  Gain 6/1 -> Mux4/1
  Demux1/2 -> Mux4/2  "q(4)"

== system test_winds/QuaternionVectorTransformation3/Quaternion Conjugate ==
  q : Inport  PortDimensions=4
  Demux : Demux  Outputs=[3 1]
  Gain : Gain  Gain=-1  SaturateOnIntegerOverflow=on  OutDataTypeStr=Inherit: Same as input  ParamDataTypeStr=Inherit: Same as input
  Mux : Mux  Inputs=2
  q' : Outport  InitialOutput=0
  wires:
  Mux/1 -> q'/1
  Demux/2 -> Mux/2  "q(4)"
  Gain/1 -> Mux/1
  Demux/1 -> Gain/1  "[ q(1)  q(2)  q(3) ]"
  q/1 -> Demux/1

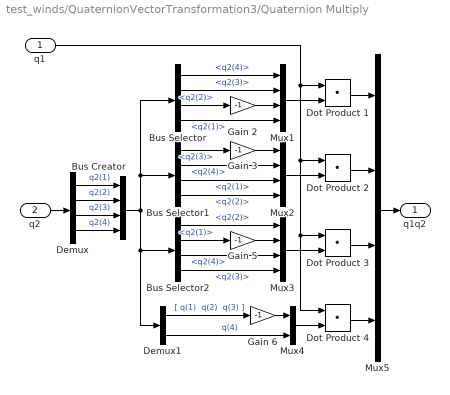
== system test_winds/QuaternionVectorTransformation3/Quaternion Multiply ==
  q1 : Inport  PortDimensions=4
  q2 : Inport  Port=2  PortDimensions=4
  Bus Creator : BusCreator
  Bus Selector : BusSelector  OutputSignals=q2(4),q2(3),q2(2),q2(1)
  Bus Selector1 : BusSelector  OutputSignals=q2(3),q2(4),q2(1),q2(2)
  Bus Selector2 : BusSelector  OutputSignals=q2(2),q2(1),q2(4),q2(3)
  Demux : Demux
  Demux1 : Demux  Outputs=[3 1]
  Dot Product {1..4} (4 alike) : DotProduct  InputSameDT=on  OutDataTypeStr=Inherit: Inherit via internal rule
  Gain {2..3,5..6} (4 alike) : Gain  Gain=-1  SaturateOnIntegerOverflow=on  OutDataTypeStr=Inherit: Same as input  ParamDataTypeStr=Inherit: Same as input
  Mux{1..3,5} (4 alike) : Mux
  Mux4 : Mux  Inputs=2
  q1q2 : Outport  InitialOutput=0
  wires:
  Demux/4 -> Bus Creator/4  "q2(4)"
  Demux/3 -> Bus Creator/3  "q2(3)"
  Demux/2 -> Bus Creator/2  "q2(2)"
  Demux/1 -> Bus Creator/1  "q2(1)"
  q2/1 -> Demux/1
  Bus Creator/1 -> Bus Selector1/1, Bus Selector/1, Bus Selector2/1, Demux1/1
  Dot Product 2/1 -> Mux5/2
  Mux5/1 -> q1q2/1
  Dot Product 4/1 -> Mux5/4
  Dot Product 3/1 -> Mux5/3
  Dot Product 1/1 -> Mux5/1
  q1/1 -> Dot Product 4/1, Dot Product 3/1, Dot Product 2/1, Dot Product 1/1
  Mux3/1 -> Dot Product 3/2
  Mux2/1 -> Dot Product 2/2
  Mux1/1 -> Dot Product 1/2
  Bus Selector2/3 -> Mux3/3  "<q2(4)>"
  Bus Selector1/2 -> Mux2/2  "<q2(4)>"
  Bus Selector/1 -> Mux1/1  "<q2(4)>"
  Bus Selector/2 -> Mux1/2  "<q2(3)>"
  Bus Selector/3 -> Gain 2/1  "<q2(2)>"
  Gain 2/1 -> Mux1/3
  Bus Selector/4 -> Mux1/4  "<q2(1)>"
  Bus Selector1/1 -> Gain 3/1  "<q2(3)>"
  Gain 3/1 -> Mux2/1
  Bus Selector1/3 -> Mux2/3  "<q2(1)>"
  Bus Selector1/4 -> Mux2/4  "<q2(2)>"
  Bus Selector2/2 -> Gain 5/1  "<q2(1)>"
  Gain 5/1 -> Mux3/2
  Bus Selector2/1 -> Mux3/1  "<q2(2)>"
  Bus Selector2/4 -> Mux3/4  "<q2(3)>"
  Mux4/1 -> Dot Product 4/2
  Demux1/1 -> Gain 6/1  "[ q(1)  q(2)  q(3) ]"
  Gain 6/1 -> Mux4/1
  Demux1/2 -> Mux4/2  "q(4)"

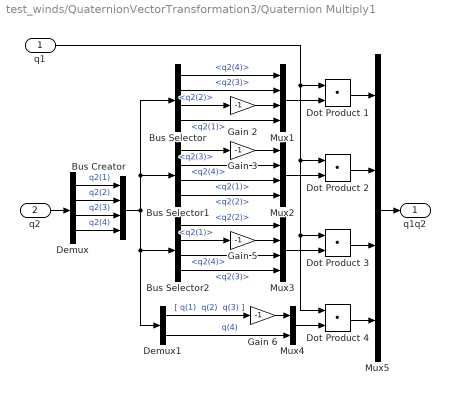
== system test_winds/QuaternionVectorTransformation3/Quaternion Multiply1 ==
  q1 : Inport  PortDimensions=4
  q2 : Inport  Port=2  PortDimensions=4
  Bus Creator : BusCreator
  Bus Selector : BusSelector  OutputSignals=q2(4),q2(3),q2(2),q2(1)
  Bus Selector1 : BusSelector  OutputSignals=q2(3),q2(4),q2(1),q2(2)
  Bus Selector2 : BusSelector  OutputSignals=q2(2),q2(1),q2(4),q2(3)
  Demux : Demux
  Demux1 : Demux  Outputs=[3 1]
  Dot Product {1..4} (4 alike) : DotProduct  InputSameDT=on  OutDataTypeStr=Inherit: Inherit via internal rule
  Gain {2..3,5..6} (4 alike) : Gain  Gain=-1  SaturateOnIntegerOverflow=on  OutDataTypeStr=Inherit: Same as input  ParamDataTypeStr=Inherit: Same as input
  Mux{1..3,5} (4 alike) : Mux
  Mux4 : Mux  Inputs=2
  q1q2 : Outport  InitialOutput=0
  wires:
  Demux/4 -> Bus Creator/4  "q2(4)"
  Demux/3 -> Bus Creator/3  "q2(3)"
  Demux/2 -> Bus Creator/2  "q2(2)"
  Demux/1 -> Bus Creator/1  "q2(1)"
  q2/1 -> Demux/1
  Bus Creator/1 -> Bus Selector1/1, Bus Selector/1, Bus Selector2/1, Demux1/1
  Dot Product 2/1 -> Mux5/2
  Mux5/1 -> q1q2/1
  Dot Product 4/1 -> Mux5/4
  Dot Product 3/1 -> Mux5/3
  Dot Product 1/1 -> Mux5/1
  q1/1 -> Dot Product 4/1, Dot Product 3/1, Dot Product 2/1, Dot Product 1/1
  Mux3/1 -> Dot Product 3/2
  Mux2/1 -> Dot Product 2/2
  Mux1/1 -> Dot Product 1/2
  Bus Selector2/3 -> Mux3/3  "<q2(4)>"
  Bus Selector1/2 -> Mux2/2  "<q2(4)>"
  Bus Selector/1 -> Mux1/1  "<q2(4)>"
  Bus Selector/2 -> Mux1/2  "<q2(3)>"
  Bus Selector/3 -> Gain 2/1  "<q2(2)>"
  Gain 2/1 -> Mux1/3
  Bus Selector/4 -> Mux1/4  "<q2(1)>"
  Bus Selector1/1 -> Gain 3/1  "<q2(3)>"
  Gain 3/1 -> Mux2/1
  Bus Selector1/3 -> Mux2/3  "<q2(1)>"
  Bus Selector1/4 -> Mux2/4  "<q2(2)>"
  Bus Selector2/2 -> Gain 5/1  "<q2(1)>"
  Gain 5/1 -> Mux3/2
  Bus Selector2/1 -> Mux3/1  "<q2(2)>"
  Bus Selector2/4 -> Mux3/4  "<q2(3)>"
  Mux4/1 -> Dot Product 4/2
  Demux1/1 -> Gain 6/1  "[ q(1)  q(2)  q(3) ]"
  Gain 6/1 -> Mux4/1
  Demux1/2 -> Mux4/2  "q(4)"

== system test_winds/QuaternionVectorTransformation4/Quaternion Conjugate ==
  q : Inport  PortDimensions=4
  Demux : Demux  Outputs=[3 1]
  Gain : Gain  Gain=-1  SaturateOnIntegerOverflow=on  OutDataTypeStr=Inherit: Same as input  ParamDataTypeStr=Inherit: Same as input
  Mux : Mux  Inputs=2
  q' : Outport  InitialOutput=0
  wires:
  q/1 -> Demux/1
  Demux/1 -> Gain/1  "[ q(1)  q(2)  q(3) ]"
  Gain/1 -> Mux/1
  Demux/2 -> Mux/2  "q(4)"
  Mux/1 -> q'/1

== system test_winds/QuaternionVectorTransformation4/Quaternion Multiply ==
  q1 : Inport  PortDimensions=4
  q2 : Inport  Port=2  PortDimensions=4
  Bus Creator : BusCreator
  Bus Selector : BusSelector  OutputSignals=q2(4),q2(3),q2(2),q2(1)
  Bus Selector1 : BusSelector  OutputSignals=q2(3),q2(4),q2(1),q2(2)
  Bus Selector2 : BusSelector  OutputSignals=q2(2),q2(1),q2(4),q2(3)
  Demux : Demux
  Demux1 : Demux  Outputs=[3 1]
  Dot Product {1..4} (4 alike) : DotProduct  InputSameDT=on  OutDataTypeStr=Inherit: Inherit via internal rule
  Gain {2..3,5..6} (4 alike) : Gain  Gain=-1  SaturateOnIntegerOverflow=on  OutDataTypeStr=Inherit: Same as input  ParamDataTypeStr=Inherit: Same as input
  Mux{1..3,5} (4 alike) : Mux
  Mux4 : Mux  Inputs=2
  q1q2 : Outport  InitialOutput=0
  wires:
  Demux1/2 -> Mux4/2  "q(4)"
  Gain 6/1 -> Mux4/1
  Demux1/1 -> Gain 6/1  "[ q(1)  q(2)  q(3) ]"
  Mux4/1 -> Dot Product 4/2
  Bus Selector2/4 -> Mux3/4  "<q2(3)>"
  Bus Selector2/1 -> Mux3/1  "<q2(2)>"
  Gain 5/1 -> Mux3/2
  Bus Selector2/2 -> Gain 5/1  "<q2(1)>"
  Bus Selector1/4 -> Mux2/4  "<q2(2)>"
  Bus Selector1/3 -> Mux2/3  "<q2(1)>"
  Gain 3/1 -> Mux2/1
  Bus Selector1/1 -> Gain 3/1  "<q2(3)>"
  Bus Selector/4 -> Mux1/4  "<q2(1)>"
  Gain 2/1 -> Mux1/3
  Bus Selector/3 -> Gain 2/1  "<q2(2)>"
  Bus Selector/2 -> Mux1/2  "<q2(3)>"
  Bus Selector/1 -> Mux1/1  "<q2(4)>"
  Bus Selector1/2 -> Mux2/2  "<q2(4)>"
  Bus Selector2/3 -> Mux3/3  "<q2(4)>"
  Mux1/1 -> Dot Product 1/2
  Mux2/1 -> Dot Product 2/2
  Mux3/1 -> Dot Product 3/2
  q1/1 -> Dot Product 1/1, Dot Product 2/1, Dot Product 3/1, Dot Product 4/1
  Dot Product 1/1 -> Mux5/1
  Dot Product 3/1 -> Mux5/3
  Dot Product 4/1 -> Mux5/4
  Mux5/1 -> q1q2/1
  Dot Product 2/1 -> Mux5/2
  Bus Creator/1 -> Demux1/1, Bus Selector2/1, Bus Selector/1, Bus Selector1/1
  q2/1 -> Demux/1
  Demux/1 -> Bus Creator/1  "q2(1)"
  Demux/2 -> Bus Creator/2  "q2(2)"
  Demux/3 -> Bus Creator/3  "q2(3)"
  Demux/4 -> Bus Creator/4  "q2(4)"

== system test_winds/QuaternionVectorTransformation4/Quaternion Multiply1 ==
  q1 : Inport  PortDimensions=4
  q2 : Inport  Port=2  PortDimensions=4
  Bus Creator : BusCreator
  Bus Selector : BusSelector  OutputSignals=q2(4),q2(3),q2(2),q2(1)
  Bus Selector1 : BusSelector  OutputSignals=q2(3),q2(4),q2(1),q2(2)
  Bus Selector2 : BusSelector  OutputSignals=q2(2),q2(1),q2(4),q2(3)
  Demux : Demux
  Demux1 : Demux  Outputs=[3 1]
  Dot Product {1..4} (4 alike) : DotProduct  InputSameDT=on  OutDataTypeStr=Inherit: Inherit via internal rule
  Gain {2..3,5..6} (4 alike) : Gain  Gain=-1  SaturateOnIntegerOverflow=on  OutDataTypeStr=Inherit: Same as input  ParamDataTypeStr=Inherit: Same as input
  Mux{1..3,5} (4 alike) : Mux
  Mux4 : Mux  Inputs=2
  q1q2 : Outport  InitialOutput=0
  wires:
  Demux1/2 -> Mux4/2  "q(4)"
  Gain 6/1 -> Mux4/1
  Demux1/1 -> Gain 6/1  "[ q(1)  q(2)  q(3) ]"
  Mux4/1 -> Dot Product 4/2
  Bus Selector2/4 -> Mux3/4  "<q2(3)>"
  Bus Selector2/1 -> Mux3/1  "<q2(2)>"
  Gain 5/1 -> Mux3/2
  Bus Selector2/2 -> Gain 5/1  "<q2(1)>"
  Bus Selector1/4 -> Mux2/4  "<q2(2)>"
  Bus Selector1/3 -> Mux2/3  "<q2(1)>"
  Gain 3/1 -> Mux2/1
  Bus Selector1/1 -> Gain 3/1  "<q2(3)>"
  Bus Selector/4 -> Mux1/4  "<q2(1)>"
  Gain 2/1 -> Mux1/3
  Bus Selector/3 -> Gain 2/1  "<q2(2)>"
  Bus Selector/2 -> Mux1/2  "<q2(3)>"
  Bus Selector/1 -> Mux1/1  "<q2(4)>"
  Bus Selector1/2 -> Mux2/2  "<q2(4)>"
  Bus Selector2/3 -> Mux3/3  "<q2(4)>"
  Mux1/1 -> Dot Product 1/2
  Mux2/1 -> Dot Product 2/2
  Mux3/1 -> Dot Product 3/2
  q1/1 -> Dot Product 1/1, Dot Product 2/1, Dot Product 3/1, Dot Product 4/1
  Dot Product 1/1 -> Mux5/1
  Dot Product 3/1 -> Mux5/3
  Dot Product 4/1 -> Mux5/4
  Mux5/1 -> q1q2/1
  Dot Product 2/1 -> Mux5/2
  Bus Creator/1 -> Demux1/1, Bus Selector2/1, Bus Selector/1, Bus Selector1/1
  q2/1 -> Demux/1
  Demux/1 -> Bus Creator/1  "q2(1)"
  Demux/2 -> Bus Creator/2  "q2(2)"
  Demux/3 -> Bus Creator/3  "q2(3)"
  Demux/4 -> Bus Creator/4  "q2(4)"

== system test_winds/cbi2LLA/-180<ang<180 ==
  In : Inport
  Degrees to Radians1 : simulink_extras/Transformations/Degrees to Radians
  Radians to Degrees : simulink_extras/Transformations/Radians to Degrees
  Trigonometric Function : Trigonometry
  Trigonometric Function1 : Trigonometry  Operator=cos
  Trigonometric Function2 : Trigonometry  Operator=atan2
  Out : Outport
  wires:
  Trigonometric Function2/1 -> Radians to Degrees/1
  In/1 -> Degrees to Radians1/1
  Trigonometric Function1/1 -> Trigonometric Function2/2
  Trigonometric Function/1 -> Trigonometric Function2/1
  Radians to Degrees/1 -> Out/1
  Degrees to Radians1/1 -> Trigonometric Function1/1, Trigonometric Function/1

== system test_winds/cbi2LLA/Subsystem ==
  P : Inport
  Q : Inport  Port=2
  Action Port : ActionPort  ActionType=else
  Constant9 : Constant  Value=3/2
  Gain1 : Gain  Gain=-1
  Gain3 : Gain  Gain=2
  Gain4 : Gain  Gain=.5
  Math Function1 : Math  Operator=sqrt  SaturateOnIntegerOverflow=on
  Math Function6 : Math  Operator=pow  SaturateOnIntegerOverflow=on
  Product1 : Product  Inputs=*/  RndMeth=Zero
  Product6 : Product  Inputs=**  RndMeth=Zero
  Trigonometric Function : Trigonometry  Operator=cos
  Trigonometric Function1 : Trigonometry  Operator=acos
  v : Outport
  wires:
  P/1 -> Gain1/1
  Gain1/1 -> Math Function1/1, Math Function6/1  "-P"
  Math Function1/1 -> Gain3/1
  Gain3/1 -> Product6/1
  Constant9/1 -> Math Function6/2
  Q/1 -> Product1/1  "Q"
  Math Function6/1 -> Product1/2
  Product1/1 -> Trigonometric Function1/1
  Trigonometric Function1/1 -> Gain4/1
  Gain4/1 -> Trigonometric Function/1
  Trigonometric Function/1 -> Product6/2
  Product6/1 -> v/1

== system test_winds/cbi2LLA/Subsystem1 ==
  D : Inport
  Q : Inport  Port=2
  Action Port : ActionPort  ActionType=then
  Constant2 : Constant  Value=1/3
  Constant3 : Constant  Value=1/3
  Math Function2 : Math  Operator=sqrt  SaturateOnIntegerOverflow=on
  Math Function3 : Math  Operator=pow  SaturateOnIntegerOverflow=on
  Math Function4 : Math  Operator=pow  SaturateOnIntegerOverflow=on
  Sum : Sum  Inputs=++|
  Sum1 : Sum  Inputs=|-+
  Sum2 : Sum  Inputs=+|-
  v : Outport
  wires:
  D/1 -> Math Function2/1  "D"
  Math Function2/1 -> Sum/1, Sum1/2
  Constant2/1 -> Math Function4/2
  Sum/1 -> Math Function4/1
  Q/1 -> Sum1/1, Sum/2  "Q"
  Constant3/1 -> Math Function3/2
  Sum1/1 -> Math Function3/1
  Math Function4/1 -> Sum2/2
  Math Function3/1 -> Sum2/1
  Sum2/1 -> v/1
